simulink model "MicroMouseTemplate0x2810x29"  (R2024a)
settings: Solver=FixedStepAuto  StartTime=0.0  StopTime=0.1  RelTol=1e-3  EnableMultiTasking=on
undefined symbols (not defined in the file): samplingTime
settings Model: STM32="{\"DigitalPortWrite\":[{\"ID\":\"MicroMouseTemplate0x2810x29:84:3\"},{\"ID\":\"MicroMouseTemplate0x2810x29:84:4\"},{\"ID\":\"MicroMouseTemplate0x2810x29:84:5\"},{\"ID\":\"MicroMouseTemplate0x2810x29:84:6\"},{\"ID\":\"MicroMouseTemplate0x2810x29:84:7\"},{\"ID\":\"MicroMouseTemplate0x2810x29:84:8\"},{\"ID\":\"MicroMouseTemplate0x2810x29:84:9\"},{\"ID\":\"MicroMouseTemplate0x2810x29:84:10\"},{\"ID\":\"MicroMouseTemplate0x2810x29:160:19\"},{\"ID\":\"MicroMouseTemplate0x2810x29:2479:4\"},{\"ID\":\"MicroMouseTemplate0x2810x29:2479:6\"},{\"ID\":\"MicroMouseTemplate0x2810x29:2479:7\"},{\"ID\":\"MicroMouseTemplate0x2810x29:2479:8\"}],\"PWMOutput\":[{\"ID\":\"MicroMouseTemplate0x2810x29:160:24\"},{\"ID\":\"MicroMouseTemplate0x2810x29:160:25\"}],\"AnalogInput\":{\"ID\":\"MicroMouseTemplate0x2810x29:2357:1\"},\"DigitalPortRead\":[{\"ID\":\"MicroMouseTemplate0x2810x29:2483:3\"},{\"ID\":\"MicroMouseTemplate0x2810x29:2483:4\"}]}"  SimulationMode=external  ExtModeTrigDuration=10  Creator=JesseJabezArendse  LastModifiedBy=sipho
settings SolverCC: AllowMultiTaskInputOutput=on  AutoInsertRateTranBlk=on  InsertRTBMode=Never (minimum delay)
settings OptimizationCC: EnhancedBackFolding=on  PassReuseOutputArgsAs=Individual arguments  StateBitsets=on  DataBitsets=on  ZeroExternalMemoryAtStartup=off  ZeroInternalMemoryAtStartup=off  NoFixptDivByZeroProtection=on  MaxStackSize=64  OptimizeBlockOrder=speed  DifferentSizesBufferReuse=on  EfficientTunableParamExpr=on
settings DebuggingCC: MultiTaskCondExecSysMsg=none  ParameterOverflowMsg=none  ParameterPrecisionLossMsg=none  ParameterTunabilityLossMsg=error
settings HardwareCC: ProdBitPerPointer=32  ProdBitPerSizeT=32  ProdBitPerPtrDiffT=32  ProdLargestAtomicInteger=Long  ProdLargestAtomicFloat=Double  ProdWordSize=32  ProdLongLongMode=on  ProdHWDeviceType=ARM Compatible->ARM Cortex  TargetBitPerPointer=64  TargetBitPerSizeT=64  TargetBitPerPtrDiffT=64  TargetLongLongMode=on  TargetIntDivRoundTo=Zero  TargetEndianess=LittleEndian  TargetWordSize=64  TargetHWDeviceType=MATLAB Host
settings ModelReferenceCC: EnableParallelModelReferenceBuilds=on  ParallelModelReferenceMATLABWorkerInit=Copy Base Workspace  SupportModelReferenceSimTargetCustomCode=on
settings SFSimCC: MATLABDynamicMemAlloc=off  SimHardwareAcceleration=native
settings RTWCC: Description=Embedded Coder  SystemTargetFile=ert.tlc  HardwareBoard=STM32L4xx Based  TLCOptions=-p0 -aInlineSetEventsForThisBaseRateFcn=TLC_FALSE -aSuppressMultiTaskScheduler=TLC_FALSE -aRateBasedStepFcn=1  TemplateMakefile=ert_default_tmf  Toolchain=GNU Tools for ARM Embedded Processors  CodeExecutionProfiling=on  CodeProfilingInstrumentation=coarse  GPUComputeCapability=3.5
settings RTWCC: CustomHeaderCode=|
  | #include "MicroMouseProgramming\Core\Inc\IMU.h"
  | #include "MicroMouseProgramming\Core\Inc\CustomWhile.h"
  | #include "MicroMouseProgramming\Core\Inc\Motors.h"
settings RTWCC: CustomInclude=|
  | MicroMouseProgramming\Core\Inc\
  | MicroMouseProgramming\Core\Src\
settings RTWCC: CustomSource=|
  | MicroMouseProgramming\Core\Src\IMU.c
  | MicroMouseProgramming\Core\Src\CustomWhile.c
  | MicroMouseProgramming\Core\Src\Motors.c
settings CodeAppCC: ForceParamTrailComments=on  IgnoreCustomStorageClasses=off  OperatorAnnotations=on  SimulinkDataObjDesc=on  SFDataObjDesc=on  InsertBlockDesc=on
settings ERTTargetCC: CodeReplacementLibrary=ARM Cortex-M  SupportNonFinite=off  SupportComplex=off  SupportContinuousTime=on  ExtModeTransport=3  ExtModeStaticAlloc=on  ExtModeStaticAllocSize=2048  ExtModeMexFile=ext_xcp  ExtModeIntrfLevel=Level2 - Open

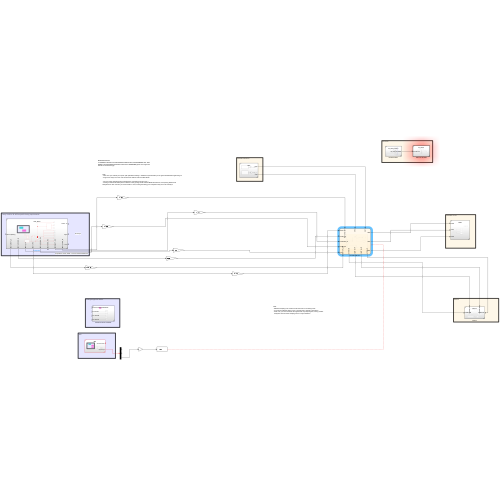
[thumbnail: Simulink's stored preview of the top-level diagram]
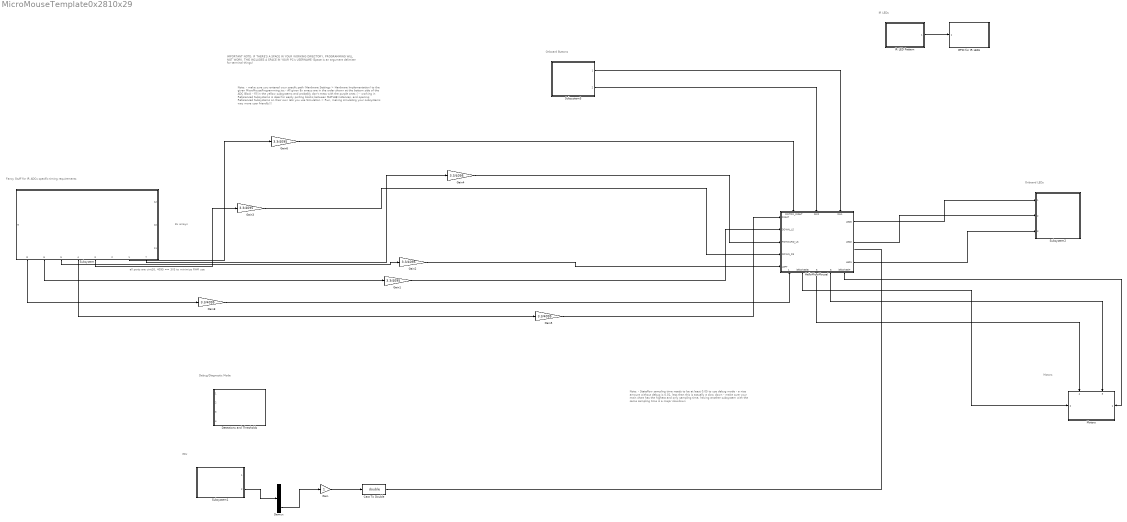
== system MicroMouseTemplate0x2810x29 ==
  note: IMPORTANT NOTE:
      | IF THERE'S A SPACE IN YOUR WORKING DIRECTORY, PROGRAMMING WILL NOT WORK, THIS INCLUDES A SPACE IN YOUR PC's USERNAME (Space is an argument delimiter for terminal things)
  note: Note:
      | - make sure you entered your specifc path (Hardware Settings > Hardware Implementation) to the given MicroMouseProgramming.ioc
      | - All given 8x arrays are in the order shown at the bottom side of the ADC Block
      |
      | - fill in the yellow subsystems and probably don't mess with the purple ones :)
      | - working in Referenced Subsystems is ideal for easily porting blocks between MATLAB instances, and opening Referenced Subsystems on their own lets you use Simulation > Run, making simulating your subsystems way more user friendly!!!
  note: 8x arrays
  note: all ports are uint16, 4095 == 3V3 to minimize RAM use
  note: IMU
  note: Note:
      | - Stateflow sampling time needs to be at least 0.05 to use debug mode
      | - a nice amount without debug is 0.01, less than this is actually a slow down
      | - make sure your main chart has the highest and only sampling time, having another
      | subsystem with the same sampling time is a major slowdown
  note: Fancy Stuff for IR ADCs specific timing requirements
  note: IR LEDs
  note: Motors
  note: Onboard Buttons
  note: Onboard LEDs
  note: Debug/Diagnostic Mode
  Cast To Double : DataTypeConversion  OutDataTypeStr=double  SaturateOnIntegerOverflow=off  RndMeth=Floor
  Demux : Demux  Outputs=3
  Detections and Thresholds : Subsystem  ReferencedSubsystem=DiagnosticMode
  GPIO for IR LEDs : Subsystem  TreatAsAtomicUnit=on  SystemSampleTime=samplingTime  ReferencedSubsystem=IR_LEDs
  Gain : Gain
  Gain{1..6,8} (7 alike) : Gain  Gain=3.3/4095  OutDataTypeStr=single
  HelloMicroMouse! : Stateflow chart  TreatAsAtomicUnit=on
      settings: PortSchema="{\"entries\":[{\"content\":{\"sides\":[{\"content\":{\"connectorIds\":[\"In5\",\"In9\",\"In4\",\"In6\",\"In3\"]},\"type\":\"ConnectorPlacement.EquallySpacedRectSide\",\"uuid\":\"f52daa4f-6374-42e5-9ef1-0ccc99d09b58\"},{\"content\":{\"connectorIds\":[\"Out1\",\"Out2\",\"Out3\"],\"side\":\"RIGHT\"},\"type\":\"ConnectorPlacement.EquallySpacedRectSide\",\"uuid\":\"94b478cc-4dde-45c7-a588-77cf2b43cdb7\"},{\"content\":{\"connectorIds\":[\"In2\",\"In7\",\"In8\"],\"side\":\"TOP\"},\"type\":\"ConnectorPlacement.EquallySpacedRectSide\",\"uuid\":\"afff2079-ea5c-423e-9722-09c3bbce433b\"},{\"content\":{\"connectorIds\":[\"In1\",\"Out4\",\"Out5\",\"Out6\",\"Out7\"],\"side\":\"BOTTOM\"},\"type\":\"ConnectorPlacement.EquallySpacedRectSide\",\"uuid\":\"94e93a1d-795d-41a3-b2d8-d520b2bf47ef\"}]},\"type\":\"ConnectorPlacement.EquallySpacedConnector\",\"uuid\":\"d4d35636-54af-48ac-af70-d56caef5e090\"}],\"packageUris\":[\"http://schema.mathworks.com/mf0/Connector/R2020b\"],\"version\":\"1.0\"}"
  IR LED Pattern : Subsystem  ReferencedSubsystem=IR_LED_Pattern
  Motors : Subsystem  ReferencedSubsystem=Motors
      settings: PortSchema="{\"entries\":[{\"content\":{\"sides\":[{\"content\":{\"connectorIds\":[\"In2\"]},\"type\":\"ConnectorPlacement.EquallySpacedRectSide\",\"uuid\":\"bdd6fda3-7e00-416f-94f9-e16bb6cad3a7\"},{\"content\":{\"connectorIds\":[\"In1\"],\"side\":\"RIGHT\"},\"type\":\"ConnectorPlacement.EquallySpacedRectSide\",\"uuid\":\"976ec5aa-4295-418a-9a6a-f21268880cf4\"},{\"content\":{\"connectorIds\":[\"In4\",\"In3\"],\"side\":\"TOP\"},\"type\":\"ConnectorPlacement.EquallySpacedRectSide\",\"uuid\":\"6a8d0236-ba3b-4294-b9d1-b673d9586bad\"}]},\"type\":\"ConnectorPlacement.EquallySpacedConnector\",\"uuid\":\"379a3d58-51ae-4117-a8c6-ac947241712a\"}],\"packageUris\":[\"http://schema.mathworks.com/mf0/Connector/R2020b\"],\"version\":\"1.0\"}"
  Subsystem : Subsystem  ReferencedSubsystem=ADC_Block
      settings: PortSchema="{\"entries\":[{\"content\":{\"sides\":[{\"content\":{},\"type\":\"ConnectorPlacement.EquallySpacedRectSide\",\"uuid\":\"be6b81d5-7a49-4e34-b35f-0c07892094fc\"},{\"content\":{\"connectorIds\":[\"Out7\",\"Out1\",\"Out2\",\"Out3\",\"Out4\",\"Out5\",\"Out6\",\"Out8\"],\"side\":\"RIGHT\"},\"type\":\"ConnectorPlacement.EquallySpacedRectSide\",\"uuid\":\"5e22590a-b7c0-4c63-8de4-8d81fd6c3849\"},{\"content\":{\"connectorIds\":[\"Out12\",\"Out10\",\"Out11\"],\"side\":\"TOP\"},\"type\":\"ConnectorPlacement.EquallySpacedRectSide\",\"uuid\":\"da97636e-cea0-4a10-8fe5-d807f9ee999f\"},{\"content\":{\"connectorIds\":[\"Out9\"],\"side\":\"BOTTOM\"},\"type\":\"ConnectorPlacement.EquallySpacedRectSide\",\"uuid\":\"a593d780-81a8-4730-a8bc-2bbf356cafe4\"}]},\"type\":\"ConnectorPlacement.EquallySpacedConnector\",\"uuid\":\"0bcac921-e51a-4437-9183-315712d0a8c2\"}],\"packageUris\":[\"http://schema.mathworks.com/mf0/Connector/R2020b\"],\"version\":\"1.0\"}"
  Subsystem1 : Subsystem  ReferencedSubsystem=IMU
  Subsystem2 : Subsystem  ReferencedSubsystem=LEDs
  Subsystem3 : Subsystem  ReferencedSubsystem=SWs
  wires:
  Subsystem3/1 -> HelloMicroMouse!/8(SW1)
  Subsystem3/2 -> HelloMicroMouse!/7(SW2)
  IR LED Pattern/1 -> GPIO for IR LEDs/1
  HelloMicroMouse!/1(LED0) -> Subsystem2/1
  HelloMicroMouse!/5(rightWheelF) -> Motors/4
  Gain4/1 -> HelloMicroMouse!/4(FORWARD_LS)
  Gain1/1 -> HelloMicroMouse!/9(DOWN_LS)
  HelloMicroMouse!/4(leftWheelB) -> Motors/2
  HelloMicroMouse!/6(rightWheelB) -> Motors/3
  HelloMicroMouse!/7(leftWheelF) -> Motors/1
  Gain3/1 -> HelloMicroMouse!/6(DOWN_RS)
  Subsystem/3 -> Gain3/1
  Subsystem/6 -> Gain1/1
  Subsystem/5 -> Gain2/1
  Gain2/1 -> HelloMicroMouse!/3(LEFT)
  Subsystem/4 -> Gain5/1
  Gain5/1 -> HelloMicroMouse!/5(RIGHT)
  Subsystem1/2 -> Demux/1
  Demux/3 -> Gain/1
  Gain/1 -> Cast To Double/1
  Cast To Double/1 -> ?
  HelloMicroMouse!/3(LED1) -> Subsystem2/3
  HelloMicroMouse!/2(LED2) -> Subsystem2/2
  Subsystem/7 -> Gain4/1
  Subsystem/1 -> Gain6/1
  Gain6/1 -> HelloMicroMouse!/2(MOTOR_RIGHT)
  Subsystem/8 -> Gain8/1
  Gain8/1 -> HelloMicroMouse!/1(MOTOR_LEFT)

== stateflow chart MicroMouseTemplate0x2810x29/HelloMicroMouse! ==
  state main
    entry:
    state UTurn
      entry,during:
      leftWheelB = 3500;
      rightWheelF = 3500;
      leftWheelF =0;
      rightWheelB =0;
    state LeftTurn
      entry,during:
      leftWheelF = 0;
      leftWheelB = 3500;
      rightWheelF = 3500;
      rightWheelB = 0;
    state IdleState
      entry:
      rightWheelB = 0;
      leftWheelB = 0;
      rightWheelF = 0;
      leftWheelF =0;
      during:
      if (RIGHT>=right)
      LED2=true;
      end
      if (LEFT>=left)
      LED0=true;
      end
      if (FORWARD_LS>=front)
      LED1=true;
      end
      if ~(RIGHT>=right)
      LED2=false;
      end
      if ~(LEFT>=left)
      LED0=false;
      end
      if ~(FORWARD_LS>=front)
      LED1=false;
      end
    state Initial
      entry:
      leftWheelB = 0;
      rightWheelB = 0;
      rightWheelF =0;
      leftWheelF =0;
    state RightTurn
      entry:
      rightWheelF =0;
      leftWheelB =0;
      rightWheelB = 4000;
      leftWheelF =4000;
    state MoveForward
      entry,during:
      rightWheelF =3500;
      rightWheelB =0;
      leftWheelF =3500;
      leftWheelB = 0;
      %code to sense walls
      if (RIGHT>=right-0.2)
      LED2=true;
      end
      if (LEFT>=left-0.2)
      LED0=true;
      end
      if (FORWARD_LS>=front*0.5)
      LED1=true;
      end
      if ~(RIGHT>=right-0.2)
      LED2=false;
      end
      if ~(LEFT>=left-0.2)
      LED0=false;
      end
      if ~(FORWARD_LS>=front*0.5)
      LED1=false;
      end
    state LineFollowing
      entry,during:
      if (DOWN_LS <= down_left)
      leftWheelB = 0;
      rightWheelF = 3500;
      leftWheelF =3000;
      rightWheelB =0;
      end
      if(DOWN_RS <down_right)
      leftWheelB = 0;
      rightWheelF = 3000;
      leftWheelF =3500;
      rightWheelB =0;
      end
    IdleState -> UTurn [order 2] : [FORWARD_LS >= front*0.5 && LEFT >=left && RIGHT >= right]
    UTurn -> IdleState : [after(1,sec)]
    LeftTurn -> IdleState : after(1,sec)
    IdleState -> LeftTurn [order 4] : [LEFT >=left  && FORWARD_LS>= front  && RIGHT < right ]
    (default) -> Initial
    Initial -> IdleState : [SW2]
    IdleState -> RightTurn [order 3] : [FORWARD_LS>=front && RIGHT>=right_threshold &&LEFT<left_threshold]
    MoveForward -> IdleState [order 1] : [MOTOR_RIGHT > motor_right && MOTOR_LEFT > motor_left ]
    IdleState -> MoveForward [order 1] : [MOTOR_RIGHT <= motor_right && MOTOR_LEFT <= motor_left]
    RightTurn -> IdleState : [after(1,sec)]
    MoveForward -> LineFollowing [order 2] : [DOWN_LS >  DOWN_RS  || DOWN_LS < DOWN_RS && FORWARD_LS<front]
    LineFollowing -> MoveForward : [after(0.1,sec)]
  state WaitUntilButtonPressed
    during:
    front = FORWARD_LS;
    left = LEFT;
    right = RIGHT;
    motor_left = MOTOR_LEFT;
    motor_right = MOTOR_RIGHT;
    down_left = DOWN_LS;
    down_right = DOWN_RS;
  (default) -> WaitUntilButtonPressed
  WaitUntilButtonPressed -> main : [SW1]
  data: MOTOR_LEFT input; MOTOR_RIGHT input; LEFT input; FORWARD_LS input; RIGHT input; DOWN_RS input; SW2 input; LED0 output; LED2 output; LED1 output; SW1 input; DOWN_LS input; leftWheelB output int16; rightWheelF output int16; rightWheelB output int16; leftWheelF output int16; left_threshold local; right_threshold local; down_rs local; down_left local; down_right local; motor_left local; motor_right local; front local; left local; right local
